simulink model "Motor_posn_model"  (R2020a)
settings: Solver=VariableStepAuto  StartTime=0.0  StopTime=10.0  RelTol=1e-3
values from neighbouring files (symbols this model uses):
  b = 3.5077E-6    [Ques_4_Parameters.sldd]
  J = 3.2284E-6    [Ques_4_Parameters.sldd]
  K = 0.0274    [Ques_4_Parameters.sldd]
  L = 2.75E-6    [Ques_4_Parameters.sldd]
  R = 4.0    [Ques_4_Parameters.sldd]
settings Model: Creator=DELL  LastModifiedBy=DELL

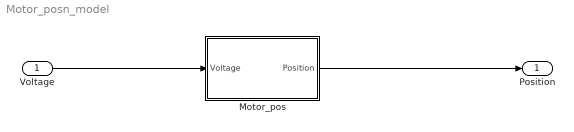
== system Motor_posn_model ==
  Voltage : Inport
  Motor_pos : Subsystem
  Position : Outport
  wires:
  Voltage/1 -> Motor_pos/1(Voltage)
  Motor_pos/1(Position) -> Position/1

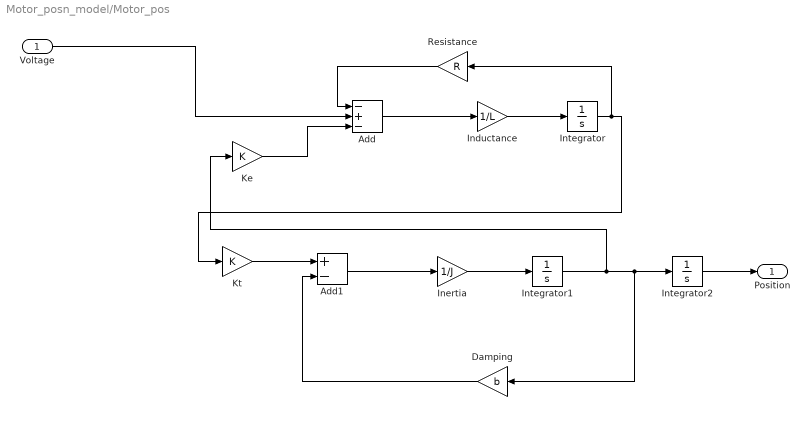
== system Motor_posn_model/Motor_pos ==
  Voltage : Inport
  Add : Sum  Inputs=-+-
  Add1 : Sum  Inputs=+-
  Damping : Gain  Gain=b
  Inductance : Gain  Gain=1/L
  Inertia : Gain  Gain=1/J
  Integrator : Integrator
  Integrator1 : Integrator
  Integrator2 : Integrator
  Ke : Gain  Gain=K
  Kt : Gain  Gain=K
  Resistance : Gain  Gain=R
  Position : Outport
  wires:
  Add1/1 -> Inertia/1
  Kt/1 -> Add1/1
  Add/1 -> Inductance/1
  Ke/1 -> Add/3
  Inductance/1 -> Integrator/1
  Integrator/1 -> Resistance/1, Kt/1
  Integrator1/1 -> Ke/1, Damping/1, Integrator2/1
  Inertia/1 -> Integrator1/1
  Resistance/1 -> Add/1
  Integrator2/1 -> Position/1
  Voltage/1 -> Add/2
  Damping/1 -> Add1/2
